simulink model "Revised_model"  (Simulink 10.3)
settings: Solver=ode3  StartTime=0.0  StopTime=12  FixedStep=ts  MaxStep=1e-4  RelTol=1e-3
undefined symbols (not defined in the file or in its folder): Ion, Lithium, sigbuilder_block, ts
libraries: spsMeanLib x9, spsSeriesRLCBranchLib x6, spsIGBTDiodeLib x4, pid_lib x4, spsPWMGeneratorDCDCLib x4, spsBatteryLib x2, spsCurrentMeasurementLib x2, spsControlledCurrentSourceLib x2, spsVoltageMeasurementLib x2, spsFirstOrderFilterLib x1, spsDiodeLib x1, spsIGBTLib x1
(part 2 of 2)

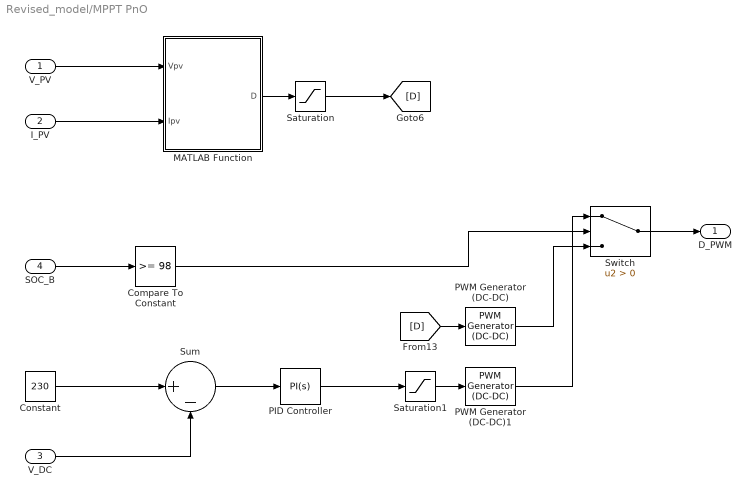
== system Revised_model/MPPT PnO ==
  V_PV : Inport
  I_PV : Inport  Port=2
  V_DC : Inport  Port=3
  SOC_B : Inport  Port=4
  Compare To Constant : simulink/Logic and Bit Operations/Compare To Constant  relop=>=  const=98  OutDataTypeStr=boolean
  Constant : Constant  Value=230
  MATLAB Function : MATLAB Function  TreatAsAtomicUnit=on
  PID Controller : pid_lib/PID Controller  Controller=PI  Form=Parallel  TimeDomain=Continuous-time  UseExternalTs=off  SampleTime=-1  IntegratorMethod=Forward Euler  FilterMethod=Forward Euler  ControllerParametersSource=internal  P=0.1  I=0.1  D=0  UseFilter=on  N=100  TunerSelectOption=Transfer Function Based (PID Tuner App)  InitialConditionSource=internal  InitialConditionForIntegrator=0  InitialConditionForFilter=0  DifferentiatorICPrevScaledInput=0  ExternalReset=none  TrackingMode=off  Kt=1  LimitOutput=off  SatLimitsSource=internal  UpperSaturationLimit=inf  LowerSaturationLimit=-inf  LinearizeAsGain=on  AntiWindupMode=none  Kb=1  POutMin=[]  POutMax=[]  IOutMin=[]  IOutMax=[]  DOutMin=[]  DOutMax=[]  NOutMin=[]  NOutMax=[]  SumOutMin=[]  SumOutMax=[]  SaturationOutMin=[]  SaturationOutMax=[]  PParamMin=[]  PParamMax=[]  IParamMin=[]  IParamMax=[]  DParamMin=[]  DParamMax=[]  NParamMin=[]  NParamMax=[]  KbParamMin=[]  KbParamMax=[]  KtParamMin=[]  KtParamMax=[]  KbOutMin=[]  KbOutMax=[]  KtOutMin=[]  KtOutMax=[]  IntegratorOutMin=[]  IntegratorOutMax=[]  FilterOutMin=[]  FilterOutMax=[]  SumI1OutMin=[]  SumI1OutMax=[]  SumI2OutMin=[]  SumI2OutMax=[]  SumI3OutMin=[]  SumI3OutMax=[]  SumI4OutMin=[]  SumI4OutMax=[]  SumDOutMin=[]  SumDOutMax=[]  DifferentiatorOutMin=[]  DifferentiatorOutMax=[]  FilterDiffOutCoefMin=[]  FilterDiffOutCoefMax=[]  ReciprocalOutMin=[]  ReciprocalOutMax=[]  SumDenOutMin=[]  SumDenOutMax=[]  SumNumOutMin=[]  SumNumOutMax=[]  DivideOutMin=[]  DivideOutMax=[]  UdiffTsProdOutMin=[]  UdiffTsProdOutMax=[]  NTsProdOutMin=[]  NTsProdOutMax=[]  UintegralTsProdOutMin=[]  UintegralTsProdOutMax=[]  UngainTsProdOutMin=[]  UngainTsProdOutMax=[]  IntegratorContinuousStateAttributes=''  IntegratorStateMustResolveToSignalObject=off  IntegratorRTWStateStorageClass=Auto  FilterContinuousStateAttributes=''  FilterStateMustResolveToSignalObject=off  FilterRTWStateStorageClass=Auto  ParallelPVariant=InternalParameters  IdealPVariant=Disabled  IVariant=InternalParameters  DVariant=Disabled  IntegratorVariant=Continuous  SatVariant=Disabled  AWVariant=Passthrough  PCopyVariant=Disabled  TRVariant=Disabled  FdbkBlocksVariant=Forward  IdealPFdbkVariant=Disabled  SatFdbkVariant=Disabled  DerivativeFilterVariant=Disabled  NVariant=Disabled  NCopyVariant=Disabled_SignalSpec  FilterICVariant=Disabled  IntegratorICVariant=InternalICs  ExternalResetVariant=Disabled  TRSumVariant=Passthrough  SumFdbkVariant=Disabled  SumVariant=Sum_PI  TsampFilterVariant=InternalTs  TsampNgainVariant=Passthrough  TsampIntegralVariant=Passthrough  ExternalSaturationOutDataTypeStr=Inherit: Same as second input
  PWM Generator (DC-DC) : spsPWMGeneratorDCDCLib/PWM Generator (DC-DC)  Fsw=5000  Ts=0
  PWM Generator (DC-DC)1 : spsPWMGeneratorDCDCLib/PWM Generator (DC-DC)  Fsw=5000  Ts=0
  Saturation : Saturate
  Saturation1 : Saturate
  Sum : Sum  Inputs=|+-
  Switch : Switch  Criteria=u2 > Threshold
  D_PWM : Outport
  wires:
  Saturation/1 -> [D]
  [D] -> PWM Generator (DC-DC)/1
  I_PV/1 -> MATLAB Function/2(Ipv)
  V_PV/1 -> MATLAB Function/1(Vpv)
  MATLAB Function/1(D) -> Saturation/1
  Sum/1 -> PID Controller/1
  V_DC/1 -> Sum/2
  Constant/1 -> Sum/1
  PID Controller/1 -> Saturation1/1
  Switch/1 -> D_PWM/1
  Saturation1/1 -> PWM Generator (DC-DC)1/1
  Compare To Constant/1 -> Switch/2
  SOC_B/1 -> Compare To Constant/1
  PWM Generator (DC-DC)/1 -> Switch/3
  PWM Generator (DC-DC)1/1 -> Switch/1

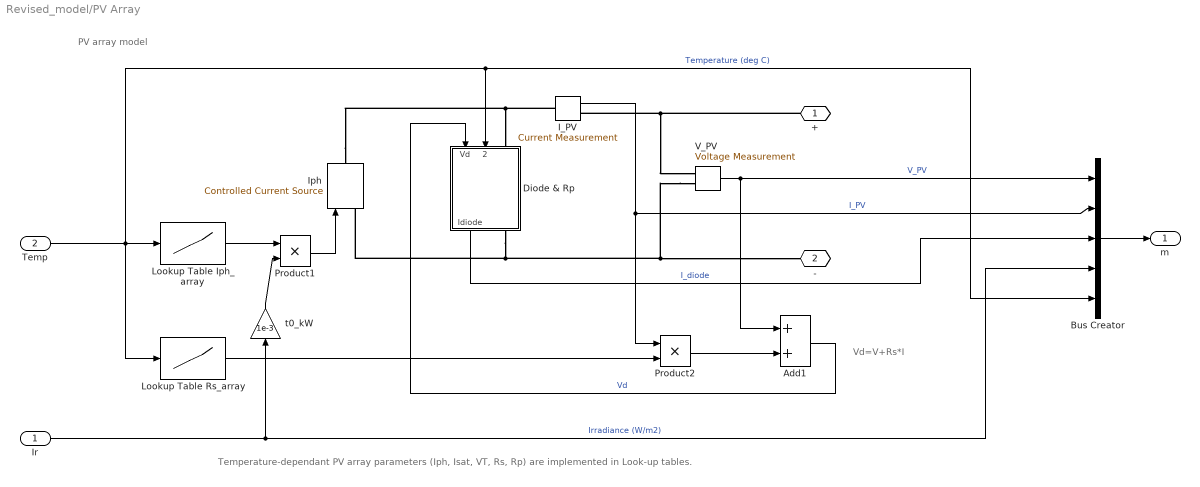
== system Revised_model/PV Array ==
  note: PV array model
  note: Vd=V+Rs*I
  note: Temperature-dependant PV array parameters (Iph, Isat, VT, Rs, Rp) are implemented in Look-up tables.
  Ir : Inport
  Temp : Inport  Port=2
  Add1 : Sum
  Bus Creator : BusCreator  Inputs=5
  Diode & Rp : Subsystem
      mask Display:
      | plot(-75,-50,100,150, [-15 -15 43 -15 -15 -75],[50 8 50 92 50 50], ...
      |     [43 43],[8 94],[100 43], [50 50])
  I_PV : spsCurrentMeasurementLib/Current Measurement  PhasorSimulation=off  OutputType=Complex  PSBequivalent=0
  Iph : spsControlledCurrentSourceLib/Controlled Current Source  Initialize=on  Source_Type=AC  Amplitude=0  Phase=0  Frequency=0  Measurements=None
  Lookup Table Iph_array : Lookup_n-D  NumberOfTableDimensions=1  BreakpointsForDimension1=TempC  Table=Iph_array  RndMeth=Simplest  InputSameDT=on
  Lookup Table Rs_array : Lookup_n-D  NumberOfTableDimensions=1  BreakpointsForDimension1=TempC  Table=Rs_array  RndMeth=Simplest  InputSameDT=on
  Product1 : Product  Inputs=**  RndMeth=Zero
  Product2 : Product  Inputs=**  RndMeth=Zero
  V_PV : spsVoltageMeasurementLib/Voltage Measurement  PhasorSimulation=off  OutputType=Complex  PSBequivalent=0
  t0_kW : Gain  Gain=1e-3
  + : PMIOPort  Side=Right
  - : PMIOPort  Port=2  Side=Right
  m : Outport
  wires:
  Bus Creator/1 -> m/1
  Lookup Table Rs_array/1 -> Product2/2
  Lookup Table Iph_array/1 -> Product1/1
  Temp/1 -> Lookup Table Iph_array/1, Diode & Rp/2(TempC), Bus Creator/5, Lookup Table Rs_array/1  "Temperature (deg C)"
  Product1/1 -> Iph/1
  Ir/1 -> Bus Creator/4, t0_kW/1  "Irradiance (W/m2)"
  I_PV/1 -> Bus Creator/2, Product2/1  "I_PV"
  t0_kW/1 -> Product1/2
  Diode & Rp/1(Idiode) -> Bus Creator/3  "I_diode"
  V_PV/1 -> Bus Creator/1, Add1/1  "V_PV"
  Product2/1 -> Add1/2
  Add1/1 -> Diode & Rp/1(Vd)  "Vd"
  connections:
  V_PV/LConn2 -- Diode & Rp/RConn1 -- Iph/LConn1 -- -/RConn1
  Iph/RConn1 -- I_PV/LConn1 -- Diode & Rp/LConn1
  +/RConn1 -- I_PV/RConn1 -- V_PV/LConn1

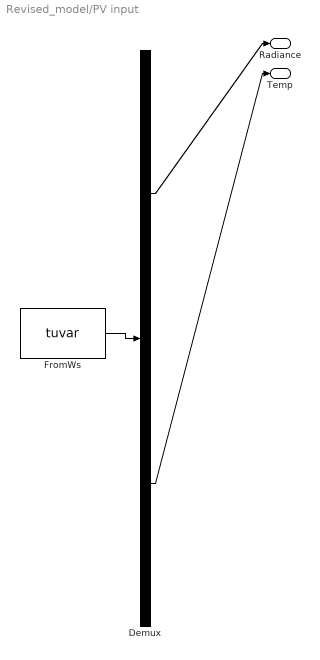
== system Revised_model/PV input ==
  Demux : Demux  Tag=STV Demux  Outputs=2
      settings: DisplayOption=none
  FromWs : FromWorkspace  Tag=STV FromWs  VariableName=tuvar  SigBuilderData=DataTag0  VnvData=DataTag1
      SigBuilderData=|
      | common.afterFinalStr = 'Extrapolate'
      | common.sampleTime = 0
      | dataSet.timeRange = [0 12]
      | dataSet.name = 'Imported_Group 1'
      | sbobj.Name = 'Signal Builder'
      | sbobj.Groups.Name = 'Imported_Group 1'
      | sbobj.Groups.Signals(1).Name = 'Radiance'
      | sbobj.Groups.Signals(1).XData = [0 1 1.001 2 2.001 3 3.001 4 4.001 5 5.001 6 6.001 7 7.001 8 8.001 9 9.001 10 10.001 11 11.001 12]
      | sbobj.Groups.Signals(1).YData = [178.5 178.5 384.69 384.69 594.38 594.38 785.89 785.89 934.7 934.7 1000 1000 1000 1000 998.89 1000 873.03 873.03 693.5 693.5 493.88 493.88 280.78 280.78]
      | sbobj.Groups.Signals(2).Name = 'Temp'
      | sbobj.Groups.Signals(2).XData = [0 1 1.001 2 2.001 3 3.001 4 4.001 5 5.001 6 6.001 7 7.001 8 8.001 9 9.001 10 10.001 11 11.001 12]
      | sbobj.Groups.Signals(2).YData = [9.27 9.27 10.18 10.18 13 13 14 14 16 16 17 17 19 19 20 20 21 21 21 21 21 21 21 21]
      | sbobj.Groups.TimeRange = [0 12]
  Radiance : Outport  Tag=STV Outport
  Temp : Outport  Tag=STV Outport  Port=2
  wires:
  FromWs/1 -> Demux/1
  Demux/1 -> Radiance/1
  Demux/2 -> Temp/1

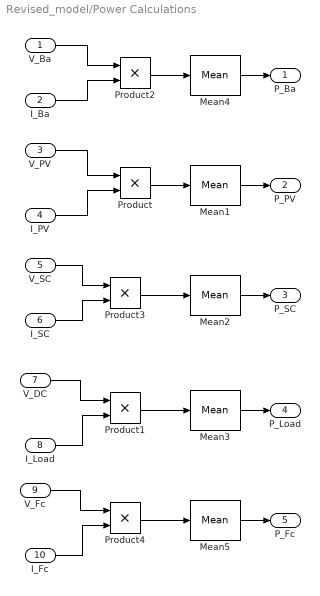
== system Revised_model/Power Calculations ==
  V_Ba : Inport
  I_Ba : Inport  Port=2
  V_PV : Inport  Port=3
  I_PV : Inport  Port=4
  V_SC : Inport  Port=5
  I_SC : Inport  Port=6
  V_DC : Inport  Port=7
  I_Load : Inport  Port=8
  V_Fc : Inport  Port=9
  I_Fc : Inport  Port=10
  Mean{1..5} (5 alike) : spsMeanLib/Mean  Freq=60  Vinit=0  Ts=0
  Product{,1..4} (5 alike) : Product
  P_Ba : Outport
  P_PV : Outport  Port=2
  P_SC : Outport  Port=3
  P_Load : Outport  Port=4
  P_Fc : Outport  Port=5
  wires:
  I_Ba/1 -> Product2/2
  V_Ba/1 -> Product2/1
  V_PV/1 -> Product/1
  I_PV/1 -> Product/2
  V_DC/1 -> Product1/1
  I_Load/1 -> Product1/2
  V_SC/1 -> Product3/1
  I_SC/1 -> Product3/2
  Mean4/1 -> P_Ba/1
  Product2/1 -> Mean4/1
  Mean1/1 -> P_PV/1
  Product/1 -> Mean1/1
  Mean2/1 -> P_SC/1
  Product3/1 -> Mean2/1
  Mean3/1 -> P_Load/1
  Product1/1 -> Mean3/1
  Product4/1 -> Mean5/1
  Mean5/1 -> P_Fc/1
  I_Fc/1 -> Product4/2
  V_Fc/1 -> Product4/1

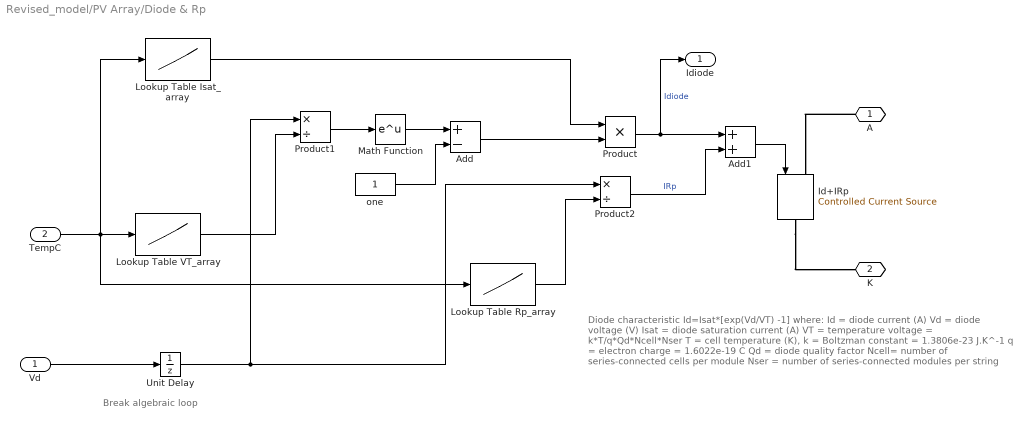
== system Revised_model/PV Array/Diode & Rp ==
  note: Diode characteristic
      |    Id=Isat*[exp(Vd/VT) -1]
      |
      | where:
      |    Id = diode current (A)
      |    Vd = diode voltage (V)
      |  Isat = diode saturation current (A)
      |    VT = temperature voltage = k*T/q*Qd*Ncell*Nser
      |     T = cell temperature (K),
      |     k = Boltzman constant = 1.3806e-23 J.K^-1
      |     q = electron charge = 1.6022e-19 C
      |    Qd = diode quality factor
      |  Ncell= number of series-connected cells per module
      |  Nser = number of series-connected modules per string
  note: Break algebraic loop
  Vd : Inport
  TempC : Inport  Port=2
  Add : Sum  Inputs=+-
  Add1 : Sum
  Id+IRp : spsControlledCurrentSourceLib/Controlled Current Source  Initialize=on  Source_Type=AC  Amplitude=0  Phase=0  Frequency=0  Measurements=None
  Lookup Table Isat_array : Lookup_n-D  NumberOfTableDimensions=1  BreakpointsForDimension1=TempC  Table=Isat_array  RndMeth=Simplest  InputSameDT=on
  Lookup Table Rp_array : Lookup_n-D  NumberOfTableDimensions=1  BreakpointsForDimension1=TempC  Table=Rp_array  RndMeth=Simplest  InputSameDT=on
  Lookup Table VT_array : Lookup_n-D  NumberOfTableDimensions=1  BreakpointsForDimension1=TempC  Table=VT_array  RndMeth=Simplest  InputSameDT=on
  Math Function : Math  SignedPower=on  SaturateOnIntegerOverflow=on
  Product : Product  RndMeth=Zero
  Product1 : Product  Inputs=*/  RndMeth=Zero
  Product2 : Product  Inputs=*/  RndMeth=Zero
  Unit Delay : UnitDelay  SampleTime=Ts  HasFrameUpgradeWarning=on
  one : Constant
  A : PMIOPort  Side=Left
  K : PMIOPort  Port=2  Side=Right
  Idiode : Outport
  wires:
  Lookup Table Rp_array/1 -> Product2/2
  Lookup Table Isat_array/1 -> Product/1
  TempC/1 -> Lookup Table Rp_array/1, Lookup Table VT_array/1, Lookup Table Isat_array/1
  Lookup Table VT_array/1 -> Product1/2
  Add/1 -> Product/2
  one/1 -> Add/2
  Product1/1 -> Math Function/1
  Product/1 -> Idiode/1, Add1/1  "Idiode"
  Vd/1 -> Unit Delay/1
  Product2/1 -> Add1/2  "IRp"
  Add1/1 -> Id+IRp/1
  Unit Delay/1 -> Product2/1, Product1/1
  Math Function/1 -> Add/1
  connections:
  A/RConn1 -- Id+IRp/LConn1
  Id+IRp/RConn1 -- K/RConn1

== matlab function MPPT PnO/MATLAB Function ==
  settings: updateMethod=DISCRETE  sampleTime=1e-4
  data: Vpv input double; D output double; Ipv input double
function D = PandO(Vpv,Ipv)

persistent Dold Pold Vold


if isempty(Dold)
    Dold = 0.35;
    Vold = 17;
    Pold = 120;
end


deltaD = 0.001;

Ppv = Vpv*Ipv;

if (Ppv-Pold) ~= 0
    if (Ppv-Pold) > 0
        if (Vpv-Vold) > 0
            D = Dold - deltaD;
        else
            D = Dold + deltaD;
        end
    else
        if (Vpv-Vold) > 0
            D = Dold + deltaD;
        else
            D = Dold - deltaD;
        end        
    end
else
    D = Dold;
end

Dold = D;
Vold = Vpv;
Pold = Ppv;
